simulink model "Turbina"  (R2024a)
settings: Solver=VariableStepAuto  StartTime=0.0  StopTime=10.0  RelTol=1e-3
undefined symbols (not defined in the file): magnitude
libraries: nesl_utility x10, fl_lib x8, simulink x2, batteryecm_lib x1, spsDCMachineLib x1, ee_lib x1, spsVoltageMeasurementLib x1, sdl_lib x1, sps_lib x1
settings Model: Creator=emanuele  LastModifiedBy=emanuele

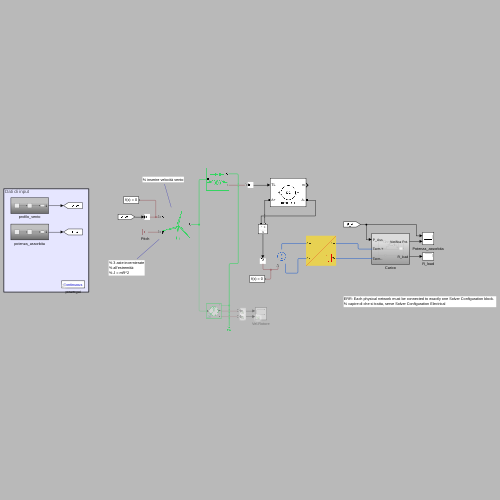
[thumbnail: Simulink's stored preview of the top-level diagram]
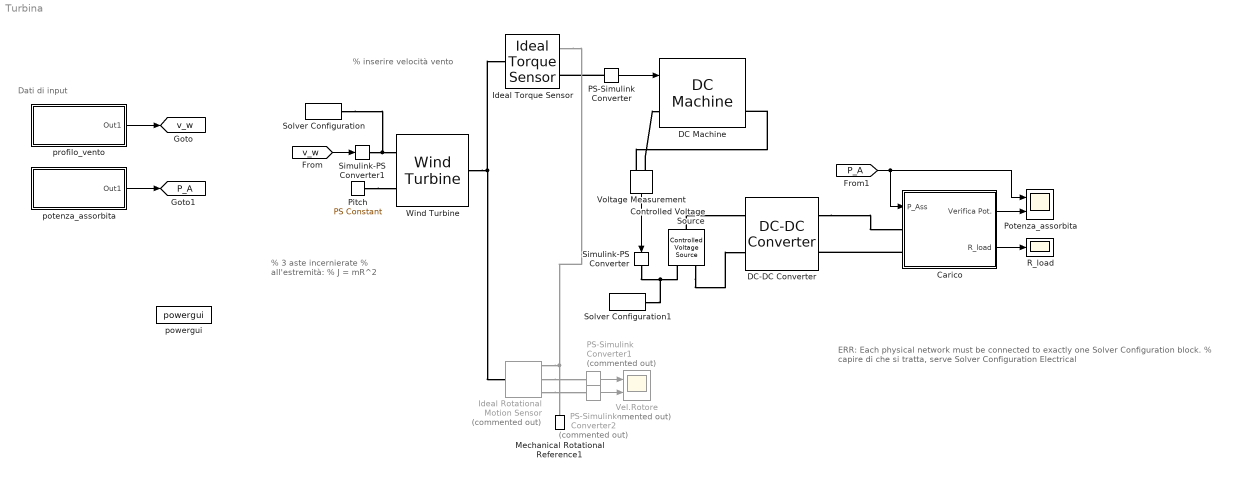
== system Turbina ==
  note: ERR: Each physical network must be connected to exactly one Solver Configuration block.
      | % capire di che si tratta, serve Solver Configuration Electrical
  note: Dati di input
  note: % inserire velocità vento
  note: % 3 aste incernierate
      | % all'estremità:
      | % J = mR^2
  Carico : Subsystem
  Controlled Voltage Source : fl_lib/Electrical/Electrical Sources/Controlled Voltage Source
  DC Machine : spsDCMachineLib/DC Machine  PresetModel=No  MechanicalLoad=Torque TL  FieldType=Permanent magnet  ShowDetailedParameters=on  MeasurementBus=off  RLa="[ 0.6  0.012]"  RLf="[ 240  120]"  Laf=1.8  MachineConstant=Torque constant (N.m/A)  Ke=1.8  Kt=1.8  J=1  Bm=0  Tf=0  w0=1  Ifinit=1  TsPowergui=0  TsBlock=-1
  DC-DC Converter : ee_lib/Semiconductors & Converters/Converters/DC-DC Converter  Vref_option=ee.enum.converters.voltageref.internal  v_ref=24 V  P_rated=1000 W  droop_enabled=true  droop_param=ee.enum.converters.droop.value  droop=0.1 V/A  droop_percent=2  Vref_droop=10 V  reversible=ee.enum.converters.directionality.unidirectional  G_diode=1e-8 1/Ohm  P_fixed=1 W  losses_option=ee.enum.converters.lossesOption.proportionalToSquaredCurrent  eff_rated=80  tableOption=ee.enum.converters.lossTableOptionThermal.currentTemp  i_eff_vec=[-2, -1, 1, 2] A  v_eff_vec=[15, 30, 45] V  eff_vec=[66, 76, 80, 74]  eff_2D_table=[66, 66, 66; 76, 76, 76; 80, 80, 80; 74, 74, 74]  model_dynamics=ee.enum.converters.dynamics.no  tau=0.02 s  v_ini=10 V  v1_min=1 V  R1=1000 Ohm  R2=1000 Ohm  enable_fault=simscape.enum.onoff.off  fault_condition=ee.enum.faults.faultInputCondition.greaterThan  fault_threshold=0.5  T_eff_vec=[280, 300, 320] K  eff_3D_table=repmat([66; 76; 80; 74], 1, 3, 3)  thermal_mass=100 J/K  initial_temperature=298.15 K
      settings: InternalSimscapePortConfiguration="{\"Bottom\":[],\"Left\":[{\"id\":\"p1\",\"label\":\"1+\",\"type\":\"foundation.electrical.electrical\"},{\"id\":\"n1\",\"label\":\"1-\",\"type\":\"foundation.electrical.electrical\"}],\"Right\":[{\"id\":\"p2\",\"label\":\"2+\",\"type\":\"foundation.electrical.electrical\"},{\"id\":\"n2\",\"label\":\"2-\",\"type\":\"foundation.electrical.electrical\"}],\"Top\":[]}"
  Ideal Rotational Motion Sensor : fl_lib/Mechanical/Mechanical Sensors/Ideal Rotational Motion Sensor  Commented=on  reference=foundation.enum.MeasurementReference.difference  acceleration_port=false  velocity_port=true  position_port=true  wrap_angle=false  offset=0 rad
  Ideal Torque Sensor : fl_lib/Mechanical/Mechanical Sensors/Ideal Torque Sensor
  Mechanical Rotational Reference1 : fl_lib/Mechanical/Rotational Elements/Mechanical Rotational Reference
  PS-Simulink Converter : nesl_utility/PS-Simulink Converter  PhysicalDomain=network_engine_domain  SubClassName=ps_output  LeftPortType=input  RightPortType=output  PseudoPeriodic=off  Frequencies=[]  VectorFormat=inherit  Unit=inherit  AffineConversion=off
  PS-Simulink Converter1 : nesl_utility/PS-Simulink Converter  Commented=on  PhysicalDomain=network_engine_domain  SubClassName=ps_output  LeftPortType=input  RightPortType=output  PseudoPeriodic=off  Frequencies=[]  VectorFormat=inherit  Unit=inherit  AffineConversion=off
  PS-Simulink Converter2 : nesl_utility/PS-Simulink Converter  Commented=on  PhysicalDomain=network_engine_domain  SubClassName=ps_output  LeftPortType=input  RightPortType=output  PseudoPeriodic=off  Frequencies=[]  VectorFormat=inherit  Unit=inherit  AffineConversion=off
  Pitch : fl_lib/Physical Signals/Sources/PS Constant  constant=3 deg
  Potenza_assorbita : Scope  NumInputPorts=2
  R_load : Scope
  Simulink-PS Converter : nesl_utility/Simulink-PS Converter  PhysicalDomain=network_engine_domain  SubClassName=ps_input  LeftPortType=input  RightPortType=output  PseudoPeriodic=off  Frequencies=[]  NoiseDistribution=none  NoiseParameters=[]  Unit=1  AffineConversion=off  FilteringAndDerivatives=provide  SimscapeFilterOrder=1  InputFilterTimeConstant=0.001  UdotUserProvided=0
  Simulink-PS Converter1 : nesl_utility/Simulink-PS Converter  PhysicalDomain=network_engine_domain  SubClassName=ps_input  LeftPortType=input  RightPortType=output  PseudoPeriodic=off  Frequencies=[]  NoiseDistribution=none  NoiseParameters=[]  Unit=1  AffineConversion=off  FilteringAndDerivatives=provide  SimscapeFilterOrder=1  InputFilterTimeConstant=0.001  UdotUserProvided=0
  Solver Configuration : nesl_utility/Solver Configuration  PhysicalDomain=network_engine_domain  SubClassName=solver  LeftPortType=input  RightPortType=generic  Tones=[]  Harmonics=[]  SimulateNoise=off  Profile=off  UseLocalSampling=off  EnableSwitchedLinearOptims=on  FrequencyDomain=off  UseCCode=off  RelTol=0.001  AbsTol=0.001  MinStep=1e-09  ToWorkspace=off  RevertToSquareIcSolve=off  NumHomotopyIterations=100  PhasorMode=off  PhasorModeNumHarmonics=1  ConsistencySolver=NEWTON_XTOL_AFTER_FTOL  IndexReductionMethod=DerivativeReplacement  DoDC=off  ResidualTolerance=1e-09  ConsistencyTolSource=GLOBAL  ConsistencyAbsTol=0.001  ConsistencyRelTol=0.001  ConsistencyTolFactor=0.001  UseLocalSolver=off  LocalSolverChoice=NE_BACKWARD_EULER_ADVANCER  ResolveIndetEquations=on  FunctionEvalNumThread=1  LocalSolverSampleTime=0.001  DoFixedCost=off  MaxNonlinIter=3  MaxModeIter=2  ComputeImpulses=off  ImpulseIterations=2  LinearAlgebra=auto  LinearAlgebraNumThread=0  EquationFormulation=NE_TIME_EF  DelaysMemoryBudget=2048  AutomaticFiltering=on  FilteringTimeConstant=0.001  PartitionStorageMethod=AS_NEEDED  PartitionMemoryBudget=1024  PartitionMethod=ROBUST  MultibodyUseLocalSolver=off  MultibodyLocalSolverChoice=ODE1  MultibodyLocalSolverSampleTime=0.001
  Solver Configuration1 : nesl_utility/Solver Configuration  PhysicalDomain=network_engine_domain  SubClassName=solver  LeftPortType=input  RightPortType=generic  Tones=[]  Harmonics=[]  SimulateNoise=off  Profile=off  UseLocalSampling=off  EnableSwitchedLinearOptims=on  FrequencyDomain=off  UseCCode=off  RelTol=0.001  AbsTol=0.001  MinStep=1e-09  ToWorkspace=off  RevertToSquareIcSolve=off  NumHomotopyIterations=100  PhasorMode=off  PhasorModeNumHarmonics=1  ConsistencySolver=NEWTON_XTOL_AFTER_FTOL  IndexReductionMethod=DerivativeReplacement  DoDC=off  ResidualTolerance=1e-09  ConsistencyTolSource=GLOBAL  ConsistencyAbsTol=0.001  ConsistencyRelTol=0.001  ConsistencyTolFactor=0.001  UseLocalSolver=off  LocalSolverChoice=NE_BACKWARD_EULER_ADVANCER  ResolveIndetEquations=on  FunctionEvalNumThread=1  LocalSolverSampleTime=0.001  DoFixedCost=off  MaxNonlinIter=3  MaxModeIter=2  ComputeImpulses=off  ImpulseIterations=2  LinearAlgebra=auto  LinearAlgebraNumThread=0  EquationFormulation=NE_TIME_EF  DelaysMemoryBudget=2048  AutomaticFiltering=on  FilteringTimeConstant=0.001  PartitionStorageMethod=AS_NEEDED  PartitionMemoryBudget=1024  PartitionMethod=ROBUST  MultibodyUseLocalSolver=off  MultibodyLocalSolverChoice=ODE1  MultibodyLocalSolverSampleTime=0.001
  Vel.Rotore : Scope  Commented=on  NumInputPorts=2
  Voltage Measurement : spsVoltageMeasurementLib/Voltage Measurement  PhasorSimulation=off  OutputType=Complex  PSBequivalent=0
  Wind Turbine : sdl_lib/Engines & Motors/Wind Turbine  parameterization=sdl.enum.WindTurbineParameterization.PowerThrust  R_rotor=90 cm  pitch_TLU=[0, 3, 5, 10, 20, 90] deg  lambda_TLU=[0, 2, 4, 6, 8, 10, 12, 14, 15]  Cp_TLU=[0.0010, 0.0161, 0.1446, 0.3865, 0.5009, 0.4404, 0.2545, 0.0002, -0.1384; 0.0016, 0.0173, 0.1079, 0.2676, 0.3779, 0.4111, 0.3838, 0.3176, 0.2753; 0.0027, 0.0197, 0.1151, 0.2606, 0.3469, 0.3558, 0.3069, 0.2222, 0.1718; 0.0054, 0.0283, 0.1315, 0.2364, 0.2589, 0.2022, 0.0929, -0.0455, -0.1204; 0.0109, 0.0536, 0.1320, 0.1256, 0.0120, -0.1752, -0.4017, -0.6435, -0.7655; -0.01 * ones(1, 9)]  Ct_TLU=[0.0000, 0.2451, 0.6740, 0.9616, 1.0000, 0.9882, 0.8430, 0.0002, -0.1341; 0.0016, 0.2541, 0.5942, 0.8582, 0.9561, 0.9754, 0.9599, 0.9092, 0.8669; 0.0027, 0.2705, 0.6113, 0.8503, 0.9339, 0.9407, 0.8993, 0.8016, 0.7239; 0.0054, 0.3215, 0.6475, 0.8205, 0.8482, 0.7727, 0.5565, -0.0450, -0.1171; 0.2035, 0.4335, 0.6485, 0.6348, 0.2129, -0.1684, -0.3701, -0.5712, -0.6681; -0.05 * ones(1, 9)]  n_blades=3  radial_TLU=[.1, .17, .23, .36, .5, .63, 1]  twist_TLU=[13.31, 13.31, 11.48, 9.01, 6.54, 4.19, .11] deg  chord_TLU=[.068, .074, .076, .069, .061, .053, .023]  alpha_TLU=[-180 : 10 : 180] deg  Cl_TLU=[0, 0, 0, 0, 0, 0, 0; 0, .397, .547, .547, .735, .788, .749; 0, .642, .685, .685, .695, .67, .659; 0, .757, .816, .816, .828, .797, .783; 0, .762, .832, .832, .846, .813, .798; 0, .68, .756, .756, .771, .739, .724; 0, .532, .609, .609, .624, .596, .581; 0, .337, .411, .411, .426, .403, .39; 0, .114, .182, .182, .195, .179, .169; 0, -.12, -.061, -.061, -.05, -.06, -.067; 0, -.349, -.302, -.302, -.294, -.295, -.299; 0, -.557, -.523, -.523, -.518, -.512, -.512; 0, -.727, -.708, -.708, -.706, -.693, -.689; 0, -.842, -.838, -.838, -.839, -.82, -.814; 0, -.886, -.895, -.895, -.898, -.875, -.866; 0, -.839, -.858, -.858, -.862, -.838, -.829; 0, -.685, -1.013, -1.013, -.815, -.869, -.958; 0, -.311, -.8496, -.8496, -.8284, -.8284, -.711; 0, .137, .288, .288, .444, .521, .442; 0, 1.368, 1.458, 1.458, 1.442, 1.358, 1.382; 0, 1.7825, 1.398, 1.398, 1.354, 1.311, 1.428; 0, 1.904, 1.265, 1.265, 1.076, .962, .926; 0, 1.903, 1.258, 1.258, 1.064, .95, .804; 0, 1.69, 1.146, 1.146, .98, .884, .763; 0, 1.323, .932, .932, .81, .74, .656; 0, .88, .657, .657, .582, .54, .495; 0, .449, .362, .362, .326, .304, .291; 0, .124, .092, .092, .072, .053, .053; 0, -.118, -.15, -.15, -.17, -.198, -.199; 0, -.348, -.379, -.379, -.399, -.434, -.436; 0, -.549, -.578, -.578, -.596, -.637, -.64; 0, -.702, -.727, -.727, -.743, -.787, -.79; 0, -.787, -.807, -.807, -.821, -.864, -.868; 0, -.782, -.797, -.797, -.806, -.847, -.85; 0, -.664, -.673, -.673, -.679, -.711, -.714; 0, -.41, -.547, -.547, -.735, -.788, -.749; 0, 0, 0, 0, 0, 0, 0]  Cd_TLU=[.35, .0602, .0267, .0267, .0202, .0185, .0198; .35, .1107, .0968, .0968, .0943, .0945, .0955; .35, .3045, .2876, .2876, .2848, .2809, .2807; .35, .5355, .5232, .5232, .5215, .5112, .5086; .35, .7685, .7656, .7656, .766, .7485, .7427; .35, .9788, .9882, .9882, .9911, .9665, .9574; .35, 1.1499, 1.173, 1.173, 1.1787, 1.1476, 1.1355; .35, 1.2716, 1.3084, 1.3084, 1.3168, 1.2805, 1.2656; .35, 1.3378, 1.3875, 1.3875, 1.3984, 1.3582, 1.341; .35, 1.346, 1.407, 1.407, 1.4201, 1.3774, 1.3587; .35, 1.2964, 1.3664, 1.3664, 1.3811, 1.3376, 1.3181; .35, 1.1918, 1.2676, 1.2676, 1.2833, 1.2409, 1.2212; .35, 1.0376, 1.1156, 1.1156, 1.1315, 1.0919, 1.0731; .35, .8429, .9187, .9187, .9341, .899, .882; .35, .6215, .6904, .6904, .7042, .6754, .661; .35, .3932, .4503, .4503, .4616, .4405, .4295; .35, .1861, .2388, .2388, .2237, .1983, .1785; .35, .0931, .0718, .0718, .0287, .0287, .0111; .35, .0113, .0087, .0087, .0065, .0057, .0052; .35, .0393, .0192, .0192, .0262, .0255, .015; .35, .3998, .2689, .2689, .228, .1987, .2379; .35, .8441, .5843, .5843, .5149, .4813, .4294; .35, 1.2873, .897, .897, .7901, .7396, .6452; .35, 1.6401, 1.1686, 1.1686, 1.0378, .9781, .8664; .35, 1.836, 1.3647, 1.3647, 1.2333, 1.1796, 1.0693; .35, 1.8347, 1.4621, 1.4621, 1.3587, 1.3297, 1.2438; .35, 1.6334, 1.4544, 1.4544, 1.4063, 1.4202, 1.3809; .35, 1.3879, 1.3938, 1.3938, 1.3985, 1.4512, 1.4565; .35, 1.3795, 1.3798, 1.3798, 1.381, 1.4294, 1.4345; .35, 1.3114, 1.3063, 1.3063, 1.3041, 1.3464, 1.3512; .35, 1.1864, 1.1763, 1.1763, 1.1709, 1.2057, 1.2099; .35, 1.0102, .9962, .9962, .9883, 1.0144, 1.0179; .35, .7935, .7771, .7771, .7676, .7845, .7871; .35, .5532, .5364, .5364, .5264, .5346, .5363; .35, .3147, .3, .3, .2912, .2922, .2931; .35, .1144, .1051, .1051, .0995, .0969, .0971; .35, .0602, .0267, .0267, .0202, .0185, .0198]  n_blade_discretization=20  model_thrust=false  model_inertia=true  rotor_inertia=12.15 kg*m^2  init_rot_vel=0 rad/s  rho_air=1.225 kg/m^3  v_thr=0.1 m/s  w_thr=0.1 rad/s  root_pitch=0 deg  expose_port_C=false
      settings: InternalSimscapePortConfiguration="{\"Bottom\":[],\"Left\":[{\"id\":\"vWind\",\"label\":\"V\",\"type\":\"input\"},{\"id\":\"pitch\",\"label\":\"β\",\"type\":\"input\"}],\"Right\":[{\"id\":\"R\",\"label\":\"R\",\"type\":\"foundation.mechanical.rotational.rotational\"}],\"Top\":[]}"
  potenza_assorbita : Subsystem
  powergui : sps_lib/powergui  Priority=1  SimulationMode=Continuous  SampleTime=50e-6  frequency=60  Iterations=50  frequencyindice=0  Pbase=100e6  ErrMax=1e-4  UnitsV=kV  UnitsW=MW  buscounter=0  FunctionMessages=off  echomessages=off  EnableUseOfTLC=off  CurrentSourceSwitches=off  DisableSnubberDevices=off  DisableRonSwitches=off  DisableVfSwitches=off  DisplayEquations=off  AutomaticDiscreteSolvers=off  SolverType=Tustin/Backward Euler (TBE)  Interpol=off  ExternalGateDelay=off  methode=off  Ts=100  x0status=blocks  SPID=on  SwTol=0  HookPort=off  NonlinearTolerance=1e-4  nMaxIteration=100  ContinueOnMaxIteration=off  RestoreLinks=warning  ResistiveCurrentMeasurement=off  Frange=[0:2:500]  Ylog=off  Xlog=on  ShowGrid=off  save=off  variable=ZData  structure=0  ZoomFFT=off  StartTime=0.0  cycles=1  DisplayStyle=1  fundamental=60  FreqAxis=off  MaxFrequency=1000  frequencyindicesteady=1  RmsSteady=1  display=off
  profilo_vento : Subsystem
  tag scope: P_A=global, v_w=global
  wires:
  Voltage Measurement/1 -> Simulink-PS Converter/1
  PS-Simulink Converter/1 -> DC Machine/1
  PS-Simulink Converter1/1 -> Vel.Rotore/1
  PS-Simulink Converter2/1 -> Vel.Rotore/2
  profilo_vento/1(Out1) -> [v_w]
  Carico/2(R_load) -> R_load/1
  Carico/1(Verifica Pot.) -> Potenza_assorbita/2
  [v_w] -> Simulink-PS Converter1/1
  potenza_assorbita/1(Out1) -> [P_A]
  [P_A] -> Potenza_assorbita/1, Carico/1(P_Ass)
  connections:
  DC-DC Converter/RConn1 -- Carico/LConn1
  Carico/LConn2 -- DC-DC Converter/RConn2
  Wind Turbine/RConn1 -- Ideal Rotational Motion Sensor/LConn1 -- Ideal Torque Sensor/LConn1
  Pitch/RConn1 -- Wind Turbine/LConn2
  Voltage Measurement/LConn1 -- DC Machine/LConn1
  Voltage Measurement/LConn2 -- DC Machine/RConn1
  Controlled Voltage Source/LConn1 -- DC-DC Converter/LConn1
  Controlled Voltage Source/RConn2 -- DC-DC Converter/LConn2
  Simulink-PS Converter/RConn1 -- Solver Configuration1/RConn1 -- Controlled Voltage Source/RConn1
  PS-Simulink Converter/LConn1 -- Ideal Torque Sensor/RConn2
  Ideal Rotational Motion Sensor/RConn2 -- PS-Simulink Converter1/LConn1
  Ideal Rotational Motion Sensor/RConn3 -- PS-Simulink Converter2/LConn1
  Simulink-PS Converter1/RConn1 -- Solver Configuration/RConn1 -- Wind Turbine/LConn1
  Ideal Rotational Motion Sensor/RConn1 -- Mechanical Rotational Reference1/LConn1 -- Ideal Torque Sensor/RConn1

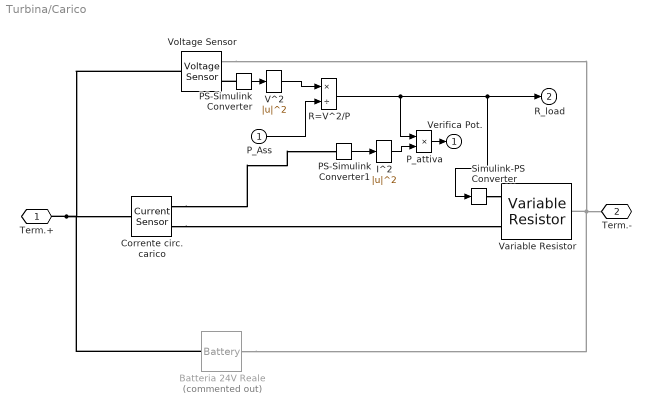
== system Turbina/Carico ==
  P_Ass : Inport  Unit=W
  Batteria 24V Reale : batteryecm_lib/Battery  Commented=on  Vnom=24 V  prm_dir=simscape.enum.battery.prm_dir.disabled  R1_dis=2 Ohm  R1_ch=2 Ohm  R1=0.5 Ohm  prm_AH=simscape.enum.battery.prm_AH.infinite  AH=50 A*hr  V1=11.5 V  AH1=25 A*hr  prm_R2=simscape.enum.battery.prm_R2.disabled  R2=2000 Ohm  Tmeas=298.15 K  charge_measurement_port=simscape.enum.battery.enable.no  prm_dyn=simscape.enum.battery.prm_dyn.off  Rp1=0.005 Ohm  tau1=30 s  Rp2=0.005 Ohm  tau2=30 s  Rp3=0.005 Ohm  tau3=30 s  Rp4=0.005 Ohm  tau4=30 s  Rp5=0.005 Ohm  tau5=30 s  prm_fade=simscape.enum.battery.prm_fade.disabled  N_fade=100  AH_fade=45 A*hr  R1_fade=2.02 Ohm  R1_ch_fade=2.02 Ohm  V1_fade=10.35 V  prm_age=simscape.enum.battery.prm_age.disabled  prm_age_OCV=simscape.enum.battery.prm_age_OCV.OCV  OCV_age=0.9  SOC_age=60  Tmeas_age=298.15 K  delta_time_age_vec=[0] d  temperature_age_vec=[273] K  OCV_scaling_age=2.2134e6  OCV_offset_age=1.632e6  temp_exp_age=0.515833569 V  t_exp_age=0.75  Vnom_T2=12 V  R1_T2=2.2 Ohm  R1_T2_dis=2.2 Ohm  R1_T2_ch=2.2 Ohm  V1_T2=11.4 V  R2_T2=2200 Ohm  Rp1_T2=0.005 Ohm  tau1_T2=30 s  Rp2_T2=0.005 Ohm  tau2_T2=30 s  Rp3_T2=0.005 Ohm  tau3_T2=30 s  Rp4_T2=0.005 Ohm  tau4_T2=30 s  Rp5_T2=0.005 Ohm  tau5_T2=30 s  Tmeas2=273.15 K  thermal_port=simscape.enum.thermaleffects.omit  thermal_mass=30000 J/K  i_specify=off  i_priority=None  i=0 A  i_nominal_specify=off  i_nominal_value=1  i_nominal_unit=A  v_specify=off  v_priority=None  v=0 V  v_nominal_specify=off  v_nominal_value=1  v_nominal_unit=V  charge_specify=off  charge_priority=High  charge=50 A*hr  charge_nominal_specify=off  charge_nominal_value=1  charge_nominal_unit=A*hr  num_cycles_specify=off  num_cycles_priority=High  num_cycles=0  num_cycles_nominal_specify=off  num_cycles_nominal_value=1  num_cycles_nominal_unit=1  temperature_specify=off  temperature_priority=High  temperature=298.15 K  temperature_nominal_specify=off  temperature_nominal_value=1  temperature_nominal_unit=K
  Corrente circ. carico : fl_lib/Electrical/Electrical Sensors/Current Sensor
      settings: SimscapeInstrumentationLogging=on
  I^2 : Math  Operator=magnitude^2
  PS-Simulink Converter : nesl_utility/PS-Simulink Converter  PhysicalDomain=network_engine_domain  SubClassName=ps_output  LeftPortType=input  RightPortType=output  PseudoPeriodic=off  Frequencies=[]  VectorFormat=inherit  Unit=inherit  AffineConversion=off
  PS-Simulink Converter1 : nesl_utility/PS-Simulink Converter  PhysicalDomain=network_engine_domain  SubClassName=ps_output  LeftPortType=input  RightPortType=output  PseudoPeriodic=off  Frequencies=[]  VectorFormat=inherit  Unit=inherit  AffineConversion=off
  P_attiva : Product
  R=V^2/P : Product  Inputs=*/
  Simulink-PS Converter : nesl_utility/Simulink-PS Converter  PhysicalDomain=network_engine_domain  SubClassName=ps_input  LeftPortType=input  RightPortType=output  PseudoPeriodic=off  Frequencies=[]  NoiseDistribution=none  NoiseParameters=[]  Unit=1  AffineConversion=off  FilteringAndDerivatives=provide  SimscapeFilterOrder=1  InputFilterTimeConstant=0.001  UdotUserProvided=0
  V^2 : Math  Operator=magnitude^2
  Variable Resistor : fl_lib/Electrical/Electrical Elements/Variable Resistor  Rmin=1 mOhm  thermalEnable=false  thermal_mass=1 J/K  i_specify=off  i_priority=None  i=0 A  i_nominal_specify=off  i_nominal_value=1  i_nominal_unit=A  v_specify=off  v_priority=None  v=0 V  v_nominal_specify=off  v_nominal_value=1  v_nominal_unit=V  T_specify=off  T_priority=None  T=300 K  T_nominal_specify=off  T_nominal_value=1  T_nominal_unit=K
  Voltage Sensor : fl_lib/Electrical/Electrical Sensors/Voltage Sensor
  Term.+ : PMIOPort  Side=Left
  Term.- : PMIOPort  Port=2  Side=Left
  Verifica Pot. : Outport
  R_load : Outport  Port=2
  wires:
  PS-Simulink Converter/1 -> V^2/1
  V^2/1 -> R=V^2/P/1
  P_Ass/1 -> R=V^2/P/2
  R=V^2/P/1 -> P_attiva/1, Simulink-PS Converter/1, R_load/1
  P_attiva/1 -> Verifica Pot./1
  PS-Simulink Converter1/1 -> I^2/1
  I^2/1 -> P_attiva/2
  connections:
  Batteria 24V Reale/RConn1 -- Voltage Sensor/RConn2 -- Variable Resistor/RConn1 -- Term.-/RConn1
  Term.+/RConn1 -- Voltage Sensor/LConn1 -- Corrente circ. carico/LConn1 -- Batteria 24V Reale/LConn1
  Corrente circ. carico/RConn2 -- Variable Resistor/LConn2
  PS-Simulink Converter/LConn1 -- Voltage Sensor/RConn1
  Corrente circ. carico/RConn1 -- PS-Simulink Converter1/LConn1
  Simulink-PS Converter/RConn1 -- Variable Resistor/LConn1

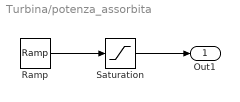
== system Turbina/potenza_assorbita ==
  Ramp : simulink/Sources/Ramp  slope=1000  start=40  InitialOutput=100
  Saturation : Saturate  UpperLimit=1000  LowerLimit=0
  Out1 : Outport
  wires:
  Ramp/1 -> Saturation/1
  Saturation/1 -> Out1/1

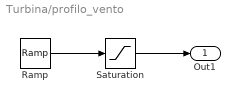
== system Turbina/profilo_vento ==
  Ramp : simulink/Sources/Ramp  slope=1  start=20  InitialOutput=10
  Saturation : Saturate  UpperLimit=15  LowerLimit=0
  Out1 : Outport
  wires:
  Saturation/1 -> Out1/1
  Ramp/1 -> Saturation/1
